simulink model "UseHWSensorData"  (R2018b)
settings: configuration reference "RPi_DynamicsRate" (kept outside this file)
values from neighbouring files (symbols this model uses):
  AccelIIR_Den = [1.000000000000000  -1.561018075800718   0.641351538057563]    [loadSensorData.m]
  AccelIIR_Num = [0.020083365564211   0.040166731128423   0.020083365564211]    [loadSensorData.m]
  M_IMU_To_Body = ZRot(pi)*EulerToDCM_321(Euler_IMU_To_Body)    [loadSensorData.m]
  NorthAngle = -84*dtr    (= -1.46607657168)    [loadSensorData.m]
  rangeTable = [2500 5000]    [loadSensorData.m]
undefined symbols (not defined in the file or in its folder): DiscIntNeverNeededParam
settings Model: Creator=barthal  LastModifiedBy=barthal
settings ConfigSetRef: SourceLocation=Base Workspace

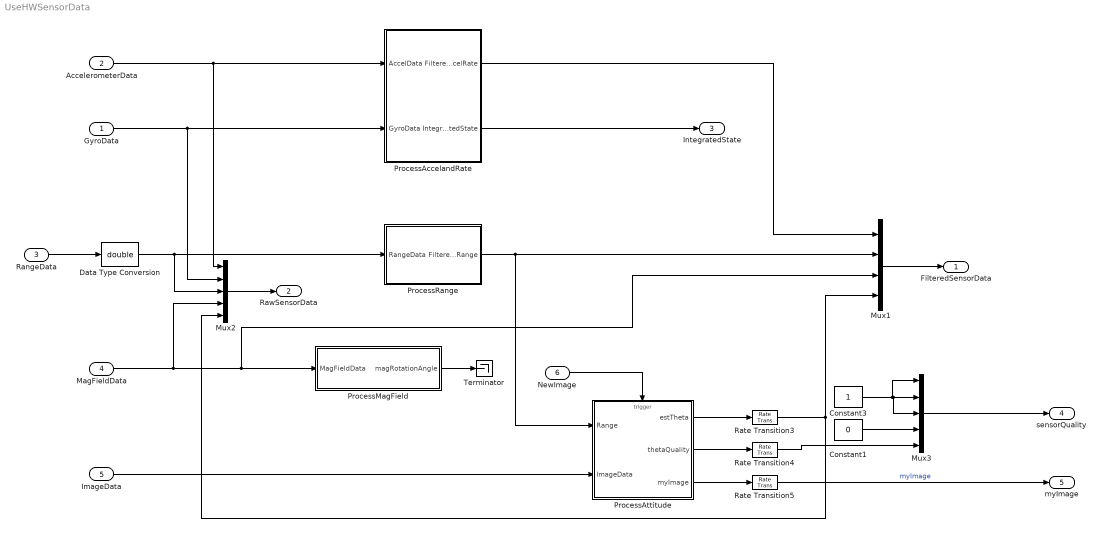
== system UseHWSensorData ==
  GyroData : Inport  PortDimensions=3
  AccelerometerData : Inport  Port=2  PortDimensions=3
  RangeData : Inport  Port=3  OutDataTypeStr=uint8  PortDimensions=4
  MagFieldData : Inport  Port=4  PortDimensions=3
  ImageData : Inport  Port=5  OutDataTypeStr=uint8
  NewImage : Inport  Port=6  OutDataTypeStr=uint8  PortDimensions=1
  Constant1 : Constant  Value=0
  Constant3 : Constant
  Data Type Conversion : DataTypeConversion  OutDataTypeStr=double
  Mux1 : Mux
  Mux2 : Mux  Inputs=5
  Mux3 : Mux  Inputs=5
  ProcessAccelandRate : Subsystem
  ProcessAttitude : Subsystem  TreatAsAtomicUnit=on
  ProcessMagField : Subsystem
  ProcessRange : Subsystem
  Rate Transition3 : RateTransition  OutPortSampleTime=dynamicsRate
  Rate Transition4 : RateTransition  OutPortSampleTime=dynamicsRate
  Rate Transition5 : RateTransition  OutPortSampleTime=dynamicsRate
  Terminator : Terminator
  FilteredSensorData : Outport
  RawSensorData : Outport  Port=2
  IntegratedState : Outport  Port=3
  sensorQuality : Outport  Port=4
  myImage : Outport  Port=5  OutDataTypeStr=uint8
  wires:
  Mux1/1 -> FilteredSensorData/1
  GyroData/1 -> Mux2/2, ProcessAccelandRate/2(GyroData)
  ProcessAccelandRate/1(FilteredAccelRate) -> Mux1/1
  AccelerometerData/1 -> Mux2/1, ProcessAccelandRate/1(AccelData)
  MagFieldData/1 -> Mux2/4, Mux1/3, ProcessMagField/1(MagFieldData)
  RangeData/1 -> Data Type Conversion/1
  Mux2/1 -> RawSensorData/1
  ProcessAccelandRate/2(IntegratedState) -> IntegratedState/1
  Constant3/1 -> Mux3/1, Mux3/3, Mux3/2
  Mux3/1 -> sensorQuality/1
  Constant1/1 -> Mux3/4
  ProcessAttitude/3(myImage) -> Rate Transition5/1
  ProcessAttitude/2(thetaQuality) -> Rate Transition4/1
  ProcessAttitude/1(estTheta) -> Rate Transition3/1
  ProcessMagField/1(magRotationAngle) -> Terminator/1
  ProcessRange/1(FilteredRange) -> ProcessAttitude/1(Range), Mux1/2
  ImageData/1 -> ProcessAttitude/2(ImageData)
  Rate Transition3/1 -> Mux2/5, Mux1/4
  Rate Transition4/1 -> Mux3/5
  Rate Transition5/1 -> myImage/1  "myImage"
  NewImage/1 -> ProcessAttitude/Trigger
  Data Type Conversion/1 -> Mux2/3, ProcessRange/1(RangeData)

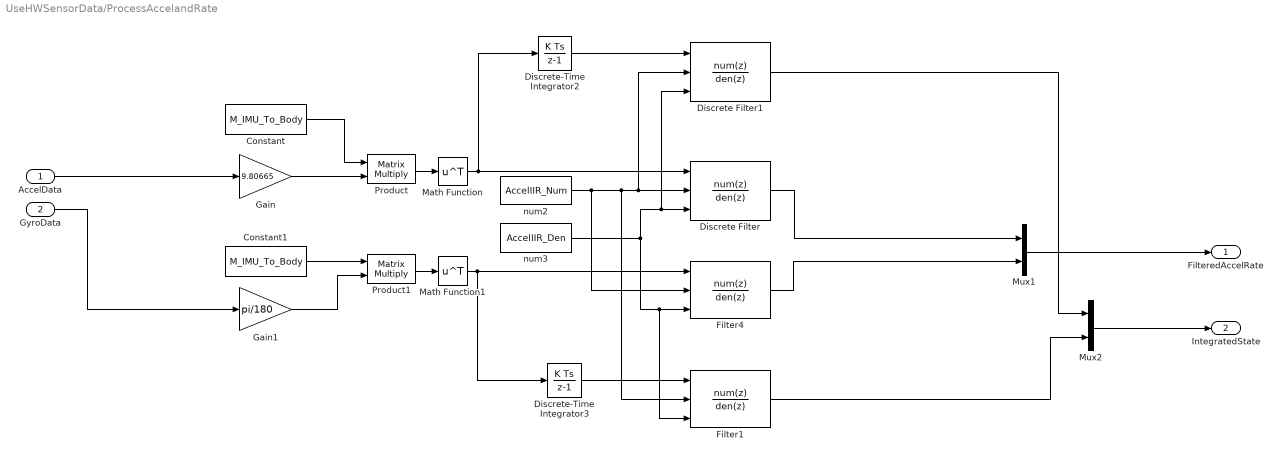
== system UseHWSensorData/ProcessAccelandRate ==
  AccelData : Inport
  GyroData : Inport  Port=2
  Constant : Constant  Value=M_IMU_To_Body
  Constant1 : Constant  Value=M_IMU_To_Body
  Discrete Filter : DiscreteFilter  NumeratorSource=Input port  DenominatorSource=Input port  a0EqualsOne=on
      settings: InputPortMap=u0,p1,p3
  Discrete Filter1 : DiscreteFilter  NumeratorSource=Input port  DenominatorSource=Input port  a0EqualsOne=on
      settings: InputPortMap=u0,p1,p3
  Discrete-Time Integrator2 : DiscreteIntegrator  SampleTime=-1  ICPrevOutput=DiscIntNeverNeededParam  ICPrevScaledInput=DiscIntNeverNeededParam
  Discrete-Time Integrator3 : DiscreteIntegrator  SampleTime=-1  ICPrevOutput=DiscIntNeverNeededParam  ICPrevScaledInput=DiscIntNeverNeededParam
  Filter1 : DiscreteFilter  Tag=BlockMethodSubSystem  NumeratorSource=Input port  Numerator=[2.46193004641406277e-06 4.92386009282812554e-06 2.46193004641406277e-06]  DenominatorSource=Input port  Denominator=[1 -1.99555712434578902 0.995566972065974776]  a0EqualsOne=on
      settings: InputPortMap=u0,p1,p3
  Filter4 : DiscreteFilter  Tag=BlockMethodSubSystem  NumeratorSource=Input port  Numerator=[2.46193004641406277e-06 4.92386009282812554e-06 2.46193004641406277e-06]  DenominatorSource=Input port  Denominator=[1 -1.99555712434578902 0.995566972065974776]  a0EqualsOne=on
      settings: InputPortMap=u0,p1,p3
  Gain : Gain  Gain=9.80665
  Gain1 : Gain  Gain=pi/180
  Math Function : Math  Operator=transpose  SaturateOnIntegerOverflow=on
  Math Function1 : Math  Operator=transpose  SaturateOnIntegerOverflow=on
  Mux1 : Mux  Inputs=2
  Mux2 : Mux  Inputs=2
  Product : Product  Multiplication=Matrix(*)
  Product1 : Product  Multiplication=Matrix(*)
  num2 : Constant  Value=AccelIIR_Num  VectorParams1D=off
  num3 : Constant  Value=AccelIIR_Den  VectorParams1D=off
  FilteredAccelRate : Outport
  IntegratedState : Outport  Port=2
  wires:
  GyroData/1 -> Gain1/1
  Product/1 -> Math Function/1
  AccelData/1 -> Gain/1
  Product1/1 -> Math Function1/1
  num3/1 -> Discrete Filter1/3, Discrete Filter/3, Filter1/3, Filter4/3
  Discrete Filter/1 -> Mux1/1
  Gain/1 -> Product/2
  Filter4/1 -> Mux1/2
  Mux1/1 -> FilteredAccelRate/1
  Constant1/1 -> Product1/1
  Gain1/1 -> Product1/2
  Constant/1 -> Product/1
  Math Function/1 -> Discrete-Time Integrator2/1, Discrete Filter/1
  Math Function1/1 -> Discrete-Time Integrator3/1, Filter4/1
  num2/1 -> Filter4/2, Filter1/2, Discrete Filter1/2, Discrete Filter/2
  Mux2/1 -> IntegratedState/1
  Discrete-Time Integrator2/1 -> Discrete Filter1/1
  Discrete Filter1/1 -> Mux2/1
  Discrete-Time Integrator3/1 -> Filter1/1
  Filter1/1 -> Mux2/2

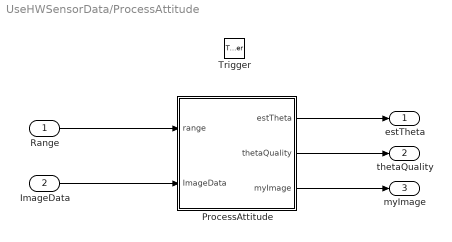
== system UseHWSensorData/ProcessAttitude ==
  Range : Inport
  ImageData : Inport  Port=2  OutDataTypeStr=uint8
  Trigger : TriggerPort  VariantControl=Variant
  ProcessAttitude : Subsystem
  estTheta : Outport
  thetaQuality : Outport  Port=2
  myImage : Outport  Port=3  OutDataTypeStr=uint8
  wires:
  Range/1 -> ProcessAttitude/1(range)
  ProcessAttitude/2(thetaQuality) -> thetaQuality/1
  ProcessAttitude/1(estTheta) -> estTheta/1
  ProcessAttitude/3(myImage) -> myImage/1
  ImageData/1 -> ProcessAttitude/2(ImageData)

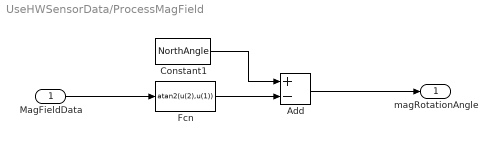
== system UseHWSensorData/ProcessMagField ==
  MagFieldData : Inport
  Add : Sum  Inputs=+-
  Constant1 : Constant  Value=NorthAngle
  Fcn : Fcn  Expr=atan2(u(2),u(1))
  magRotationAngle : Outport
  wires:
  Constant1/1 -> Add/1
  Fcn/1 -> Add/2
  MagFieldData/1 -> Fcn/1
  Add/1 -> magRotationAngle/1

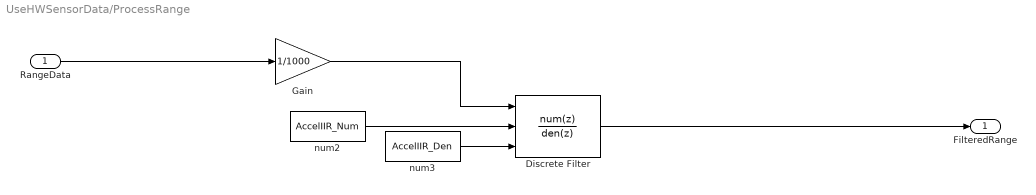
== system UseHWSensorData/ProcessRange ==
  RangeData : Inport
  Discrete Filter : DiscreteFilter  NumeratorSource=Input port  DenominatorSource=Input port  a0EqualsOne=on
      settings: InputPortMap=u0,p1,p3
  Gain : Gain  Gain=1/1000
  num2 : Constant  Value=AccelIIR_Num  VectorParams1D=off
  num3 : Constant  Value=AccelIIR_Den  VectorParams1D=off
  FilteredRange : Outport
  wires:
  num2/1 -> Discrete Filter/2
  num3/1 -> Discrete Filter/3
  RangeData/1 -> Gain/1
  Discrete Filter/1 -> FilteredRange/1
  Gain/1 -> Discrete Filter/1

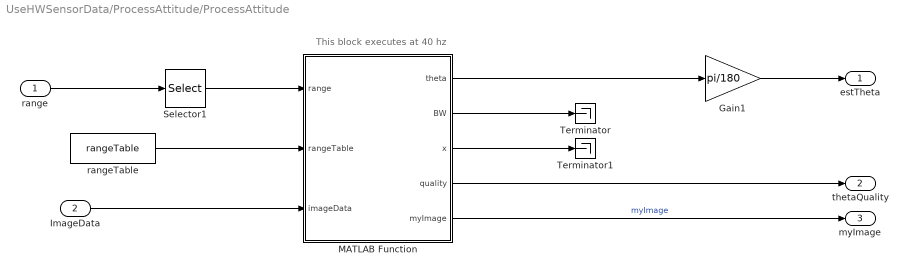
== system UseHWSensorData/ProcessAttitude/ProcessAttitude ==
  note: This block executes at 40 hz
  range : Inport  PortDimensions=4
  ImageData : Inport  Port=2  OutDataTypeStr=uint8  PortDimensions=[307200]
  Gain1 : Gain  Gain=pi/180
  MATLAB Function : MATLAB Function  TreatAsAtomicUnit=on
  Selector1 : Selector  InputPortWidth=4  IndexOptions=Index vector (dialog)  Indices=1  OutputSizes=1
  Terminator : Terminator
  Terminator1 : Terminator
  rangeTable : Constant  Value=rangeTable
  estTheta : Outport
  thetaQuality : Outport  Port=2
  myImage : Outport  Port=3  OutDataTypeStr=uint8
  wires:
  MATLAB Function/3(x) -> Terminator1/1
  MATLAB Function/2(BW) -> Terminator/1
  MATLAB Function/5(myImage) -> myImage/1  "myImage"
  MATLAB Function/4(quality) -> thetaQuality/1
  MATLAB Function/1(theta) -> Gain1/1
  range/1 -> Selector1/1
  Selector1/1 -> MATLAB Function/1(range)
  Gain1/1 -> estTheta/1
  rangeTable/1 -> MATLAB Function/2(rangeTable)
  ImageData/1 -> MATLAB Function/3(imageData)

== matlab function UseHWSensorData/ProcessAttitude/ProcessAttitude/MATLAB Function ==
  data: range input; theta output; BW output; x output; quality output; rangeTable input; imageData input; myImage output uint8
function [theta,BW,x,quality,myImage] = callimageProcess(range,rangeTable,imageData)

% persistent camObj
% 
% if isempty(camObj)
%     adaptorname = 'winvideo';
%     camObj = imaq.VideoDevice(adaptorname);
% end

% Use this if importing a 3-channel color image
% b=imageData(:,1);
% g=imageData(:,2);
% r=imageData(:,3);
% 
% b2=reshape(b,640,480);
% g2=reshape(g,640,480);
% r2=reshape(r,640,480);
% 
% myImage = uint8(zeros(480,640,3));
% 
% myImage(:,:,1) = r2';
% myImage(:,:,2) = g2';
% myImage(:,:,3) = b2';

% Use this if importing a 1 channel grayscale image
inputImage=reshape(imageData,640,480);
% myImage = uint8(zeros(480,640));
myImage = inputImage';

% theta = 0;
% BW = 0;
% x = 0;
% quality = 0;
[theta,BW,x,quality] = imageProcess(myImage,range,rangeTable);
